simulink model "Cv_bf_new_new"  (R2019b)
settings: Solver=ode4  StartTime=0.0  StopTime=0.6  FixedStep=0.00001  RelTol=1e-3
InitFcn:
  | % Paramètres de la vidéo (Test initial)
  | clc;
  | clear all;
  | 
  | Rs = 0.8;        % Résistance statorique
  | Ld = 1.1e-3;     % Inductance axe d
  | Lq = 1.32e-3;     % Inductance axe q
  | Qf= 1.5;       % Flux des aimants (Phi_f)
  | p = 2;           % Nombre de paires de pôles
  | J = 1.15e-3;     % Moment d'inertie
  | fr = 0.59e-4;     % Coefficient de frottement
libraries: simulink x1
settings Model: Creator=x1 yoga  LastModifiedBy=x1 yoga

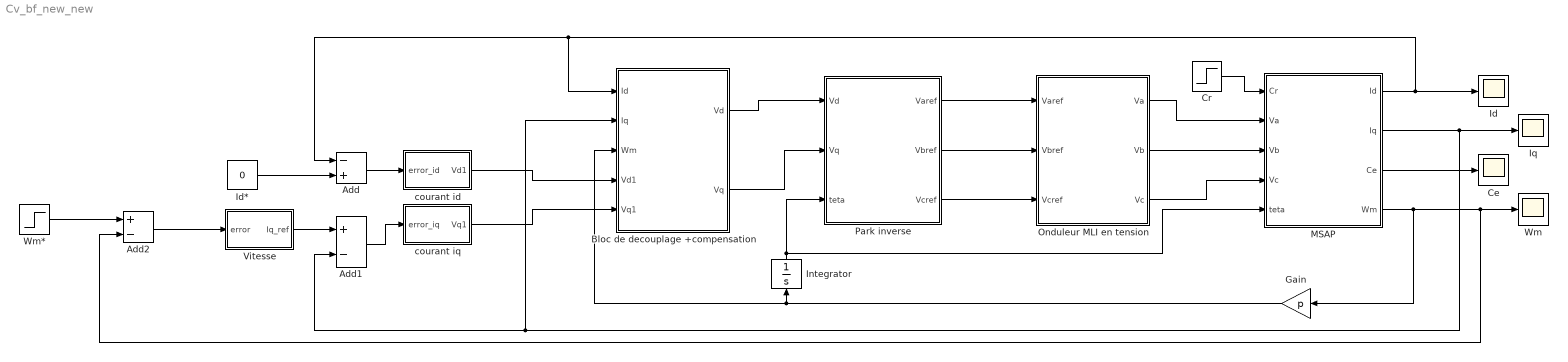
== system Cv_bf_new_new ==
  " MSAP" : Subsystem
  Add : Sum  Inputs=-+
  Add1 : Sum  Inputs=+-
  Add2 : Sum  Inputs=+-
  Bloc de decouplage +compensation : Subsystem
  Ce : Scope
  Cr : Step  Time=0.15  After=3  SampleTime=0
  Gain : Gain  Gain=p
  Id : Scope
  Id* : Constant  Value=0
  Integrator : Integrator
  Iq : Scope
  Onduleur MLI en tension : Subsystem
  Park inverse : Subsystem
  Vitesse : Subsystem  mask{Kp=50, Ki=1, Ka=150}
      mask prompts: Kp "Gain proportionnel (Kp)"; Ki "Gain intégral (Ki)"; Ka "Gain de compensation de saturation (Ka)"
      mask Display: disp('PI')
  Wm : Scope
  Wm* : Step  Time=0.3  Before=100  After=-100  SampleTime=0
  courant id : Subsystem  mask{Kp=2.56, Ki=450}
      mask prompts: Kp "Gain proportionnel (Kp)"; Ki "Gain intégral (Ki)"
      mask Display: disp('PI')
  courant iq : Subsystem  mask{Kp=2.56, Ki=450}
      mask prompts: Kp "Gain proportionnel (Kp)"; Ki "Gain intégral (Ki)"
      mask Display: disp('PI')
  wires:
  Vitesse/1(Iq_ref) -> Add1/1
  " MSAP"/3(Ce) -> Ce/1
  Id*/1 -> Add/2
  Integrator/1 -> Park inverse/3("teta "), " MSAP"/5(teta)
  " MSAP"/2(Iq) -> Bloc de decouplage +compensation/2(Iq), Add1/2, Iq/1
  Gain/1 -> Bloc de decouplage +compensation/3(Wm), Integrator/1
  Wm*/1 -> Add2/1
  " MSAP"/1(Id) -> Bloc de decouplage +compensation/1(Id), Add/1, Id/1
  Bloc de decouplage +compensation/2(Vq) -> Park inverse/2(Vq)
  Park inverse/1("Varef ") -> Onduleur MLI en tension/1(Varef)
  courant id/1(Vd1) -> Bloc de decouplage +compensation/4(Vd1)
  courant iq/1(Vq1) -> Bloc de decouplage +compensation/5(Vq1)
  Add2/1 -> Vitesse/1(error)
  Add1/1 -> courant iq/1(error_iq)
  Onduleur MLI en tension/3(Vc) -> " MSAP"/4(Vc)
  Onduleur MLI en tension/1(Va) -> " MSAP"/2(Va)
  " MSAP"/4("Wm ") -> Gain/1, Add2/2, Wm/1
  Add/1 -> courant id/1(error_id)
  Onduleur MLI en tension/2(Vb) -> " MSAP"/3(Vb)
  Park inverse/2("Vbref ") -> Onduleur MLI en tension/2(Vbref)
  Park inverse/3("Vcref ") -> Onduleur MLI en tension/3(Vcref)
  Bloc de decouplage +compensation/1(Vd) -> Park inverse/1(Vd)
  Cr/1 -> " MSAP"/1(Cr)

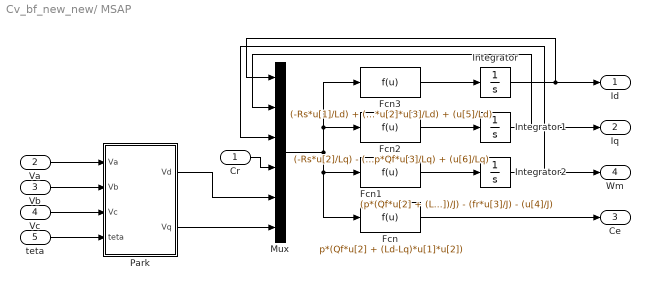
== system Cv_bf_new_new/ MSAP ==
  Cr : Inport
  Va : Inport  Port=2
  Vb : Inport  Port=3
  Vc : Inport  Port=4
  teta : Inport  Port=5
  Fcn : Fcn  Expr=p*(Qf*u[2] + (Ld-Lq)*u[1]*u[2])
  Fcn1 : Fcn  Expr=(p*(Qf*u[2] + (Ld-Lq)*u[1]*u[2])/J) - (fr*u[3]/J) - (u[4]/J)
  Fcn2 : Fcn  Expr=(-Rs*u[2]/Lq) - (p*Ld*u[3]*u[1]/Lq) - (p*Qf*u[3]/Lq) + (u[6]/Lq)
  Fcn3 : Fcn  Expr=(-Rs*u[1]/Ld) + (p*Lq*u[2]*u[3]/Ld) + (u[5]/Ld)
  Integrator : Integrator
  Integrator1 : Integrator
  Integrator2 : Integrator
  Mux : Mux  Inputs=6
  Park : Subsystem
  Id : Outport
  Iq : Outport  Port=2
  Ce : Outport  Port=3
  "Wm " : Outport  Port=4
  wires:
  Mux/1 -> Fcn1/1, Fcn/1, Fcn2/1, Fcn3/1
  Fcn/1 -> Ce/1
  Integrator1/1 -> Iq/1, Mux/2
  Vb/1 -> Park/2(Vb)
  Integrator2/1 -> "Wm "/1, Mux/3
  Integrator/1 -> Id/1, Mux/1
  Fcn2/1 -> Integrator1/1
  Park/2("Vq ") -> Mux/6
  Cr/1 -> Mux/4
  Park/1("Vd ") -> Mux/5
  Va/1 -> Park/1(Va)
  Vc/1 -> Park/3(Vc)
  Fcn3/1 -> Integrator/1
  teta/1 -> Park/4(teta)
  Fcn1/1 -> Integrator2/1

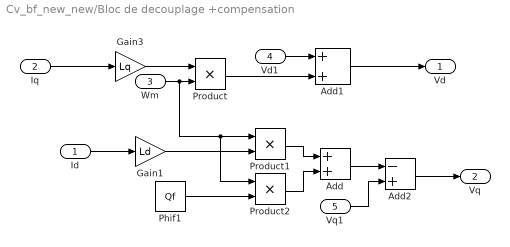
== system Cv_bf_new_new/Bloc de decouplage +compensation ==
  Id : Inport
  Iq : Inport  Port=2
  Wm : Inport  Port=3
  Vd1 : Inport  Port=4
  Vq1 : Inport  Port=5
  Add : Sum
  Add1 : Sum
  Add2 : Sum  Inputs=-+
  Gain1 : Gain  Gain=Ld
  Gain3 : Gain  Gain=Lq
  Phif1 : Constant  Value=Qf
  Product : Product
  Product1 : Product
  Product2 : Product
  Vd : Outport
  Vq : Outport  Port=2
  wires:
  Iq/1 -> Gain3/1
  Gain3/1 -> Product/1
  Wm/1 -> Product2/1, Product1/1, Product/2
  Product/1 -> Add1/2
  Vd1/1 -> Add1/1
  Add1/1 -> Vd/1
  Gain1/1 -> Product1/2
  Id/1 -> Gain1/1
  Phif1/1 -> Product2/2
  Vq1/1 -> Add2/2
  Product1/1 -> Add/1
  Product2/1 -> Add/2
  Add/1 -> Add2/1
  Add2/1 -> Vq/1

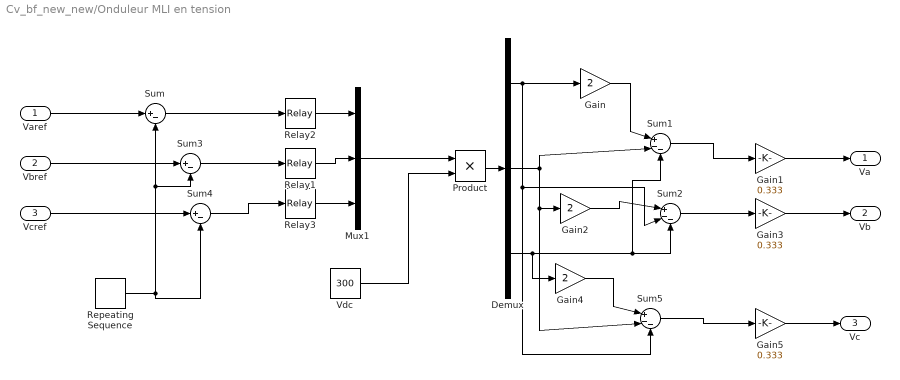
== system Cv_bf_new_new/Onduleur MLI en tension ==
  Varef : Inport
  Vbref : Inport  Port=2
  Vcref : Inport  Port=3
  Demux : Demux  Outputs=3
  Gain : Gain  Gain=2
  Gain1 : Gain  Gain=0.333
  Gain2 : Gain  Gain=2
  Gain3 : Gain  Gain=0.333
  Gain4 : Gain  Gain=2
  Gain5 : Gain  Gain=0.333
  Mux1 : Mux  Inputs=3
  Product : Product
  Relay1 : Relay
  Relay2 : Relay
  Relay3 : Relay
  Repeating Sequence : simulink/Sources/Repeating Sequence  rep_seq_t=[0 1/(2*7000) 1/7000]  rep_seq_y=[-30, 30, 30]
  Sum : Sum  Inputs=|+-
  Sum1 : Sum  Inputs=|+--
  Sum2 : Sum  Inputs=|+--
  Sum3 : Sum  Inputs=|+-
  Sum4 : Sum  Inputs=|+-
  Sum5 : Sum  Inputs=|+--
  "Vdc " : Constant  Value=300
  Va : Outport
  Vb : Outport  Port=2
  Vc : Outport  Port=3
  wires:
  Relay3/1 -> Mux1/3
  Gain4/1 -> Sum5/1
  Repeating Sequence/1 -> Sum4/2, Sum3/2, Sum/2
  Demux/1 -> Sum5/3, Sum2/2, Gain/1
  Demux/3 -> Gain4/1, Sum2/3, Sum1/3
  Sum4/1 -> Relay3/1
  Demux/2 -> Sum5/2, Gain2/1, Sum1/2
  Varef/1 -> Sum/1
  Gain2/1 -> Sum2/1
  Sum/1 -> Relay2/1
  Relay2/1 -> Mux1/1
  Sum1/1 -> Gain1/1
  Product/1 -> Demux/1
  Vcref/1 -> Sum4/1
  Sum2/1 -> Gain3/1
  Sum3/1 -> Relay1/1
  Vbref/1 -> Sum3/1
  Relay1/1 -> Mux1/2
  Sum5/1 -> Gain5/1
  Mux1/1 -> Product/1
  Gain/1 -> Sum1/1
  Gain5/1 -> Vc/1
  Gain3/1 -> Vb/1
  Gain1/1 -> Va/1
  "Vdc "/1 -> Product/2

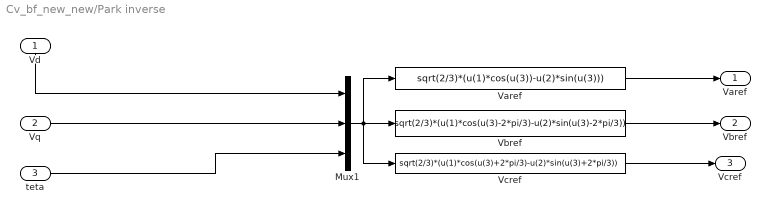
== system Cv_bf_new_new/Park inverse ==
  Vd : Inport
  Vq : Inport  Port=2
  "teta " : Inport  Port=3
  Mux1 : Mux  Inputs=3
  Varef : Fcn  Expr=sqrt(2/3)*(u(1)*cos(u(3))-u(2)*sin(u(3)))
  Vbref : Fcn  Expr=sqrt(2/3)*(u(1)*cos(u(3)-2*pi/3)-u(2)*sin(u(3)-2*pi/3))
  Vcref : Fcn  Expr=sqrt(2/3)*(u(1)*cos(u(3)+2*pi/3)-u(2)*sin(u(3)+2*pi/3))
  "Varef " : Outport
  "Vbref " : Outport  Port=2
  "Vcref " : Outport  Port=3
  wires:
  Vcref/1 -> "Vcref "/1
  Varef/1 -> "Varef "/1
  Vbref/1 -> "Vbref "/1
  Mux1/1 -> Vcref/1, Vbref/1, Varef/1
  Vd/1 -> Mux1/1
  Vq/1 -> Mux1/2
  "teta "/1 -> Mux1/3

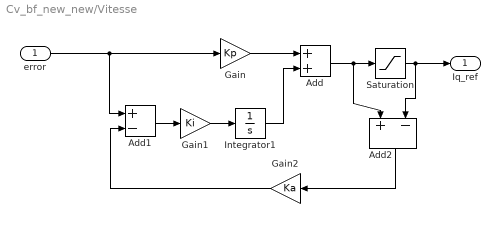
== system Cv_bf_new_new/Vitesse ==
  error : Inport
  Add : Sum
  Add1 : Sum  Inputs=+-
  Add2 : Sum  Inputs=+-
  Gain : Gain  Gain=Kp
  Gain1 : Gain  Gain=Ki
  Gain2 : Gain  Gain=Ka
  Integrator1 : Integrator
  Saturation : Saturate  UpperLimit=30  LowerLimit=-30
  Iq_ref : Outport
  wires:
  error/1 -> Add1/1, Gain/1
  Gain/1 -> Add/1
  Add/1 -> Add2/1, Saturation/1
  Gain1/1 -> Integrator1/1
  Integrator1/1 -> Add/2
  Add1/1 -> Gain1/1
  Saturation/1 -> Add2/2, Iq_ref/1
  Add2/1 -> Gain2/1
  Gain2/1 -> Add1/2

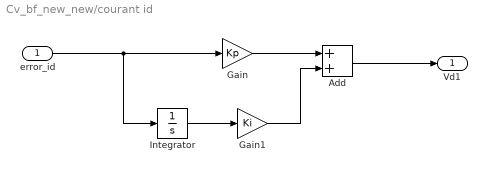
== system Cv_bf_new_new/courant id ==
  error_id : Inport
  Add : Sum
  Gain : Gain  Gain=Kp
  Gain1 : Gain  Gain=Ki
  Integrator : Integrator
  Vd1 : Outport
  wires:
  Gain1/1 -> Add/2
  error_id/1 -> Gain/1, Integrator/1
  Gain/1 -> Add/1
  Integrator/1 -> Gain1/1
  Add/1 -> Vd1/1

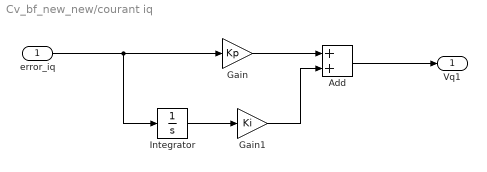
== system Cv_bf_new_new/courant iq ==
  error_iq : Inport
  Add : Sum
  Gain : Gain  Gain=Kp
  Gain1 : Gain  Gain=Ki
  Integrator : Integrator
  Vq1 : Outport
  wires:
  Gain1/1 -> Add/2
  error_iq/1 -> Gain/1, Integrator/1
  Gain/1 -> Add/1
  Integrator/1 -> Gain1/1
  Add/1 -> Vq1/1

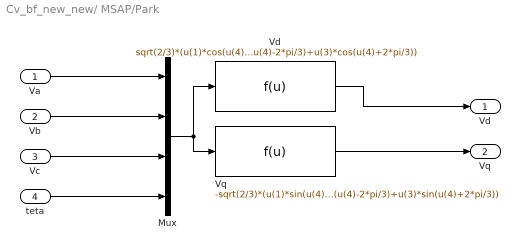
== system Cv_bf_new_new/ MSAP/Park ==
  Va : Inport
  Vb : Inport  Port=2
  Vc : Inport  Port=3
  teta : Inport  Port=4
  Mux : Mux
  Vd : Fcn  Expr=sqrt(2/3)*(u(1)*cos(u(4))+u(2)*cos(u(4)-2*pi/3)+u(3)*cos(u(4)+2*pi/3))
  Vq : Fcn  Expr=-sqrt(2/3)*(u(1)*sin(u(4))+u(2)*sin(u(4)-2*pi/3)+u(3)*sin(u(4)+2*pi/3))
  "Vd " : Outport
  "Vq " : Outport  Port=2
  wires:
  Vq/1 -> "Vq "/1
  Vd/1 -> "Vd "/1
  Vb/1 -> Mux/2
  Mux/1 -> Vq/1, Vd/1
  Va/1 -> Mux/1
  Vc/1 -> Mux/3
  teta/1 -> Mux/4
